simulink model "sensor_model"  (R2018a)
settings: Solver=VariableStepAuto  StartTime=0.0  StopTime=35  RelTol=1e-3
libraries: simulink x6
settings Model: Creator=cory0  LastModifiedBy=calvink

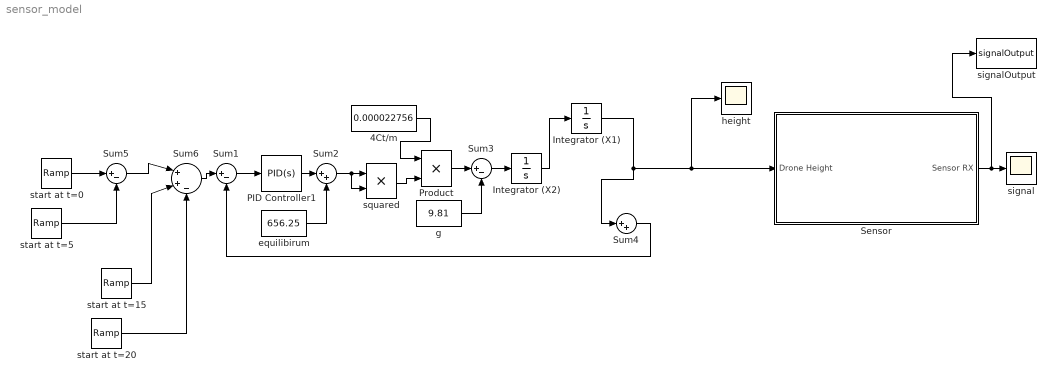
== system sensor_model ==
  4Ct/m : Constant  Value=0.000022756
  Integrator (X1) : Integrator
  Integrator (X2) : Integrator
  PID Controller1 : simulink/Continuous/PID Controller  Controller=PID  TimeDomain=Continuous-time  SampleTime=-1  IntegratorMethod=Forward Euler  FilterMethod=Forward Euler  Form=Parallel  UseFilter=on  ControllerParametersSource=internal  P=12.05  I=0  D=90  N=10  InitialConditionSource=internal  InitialConditionForIntegrator=0  InitialConditionForFilter=0  ExternalReset=none  LimitOutput=off  UpperSaturationLimit=inf  LowerSaturationLimit=-inf  LinearizeAsGain=on  AntiWindupMode=none  Kb=1  TrackingMode=off  Kt=1  PParamMin=[]  PParamMax=[]  IParamMin=[]  IParamMax=[]  DParamMin=[]  DParamMax=[]  NParamMin=[]  NParamMax=[]  KbParamMin=[]  KbParamMax=[]  KtParamMin=[]  KtParamMax=[]  POutMin=[]  POutMax=[]  IOutMin=[]  IOutMax=[]  DOutMin=[]  DOutMax=[]  NOutMin=[]  NOutMax=[]  KbOutMin=[]  KbOutMax=[]  KtOutMin=[]  KtOutMax=[]  IntegratorOutMin=[]  IntegratorOutMax=[]  FilterOutMin=[]  FilterOutMax=[]  SumOutMin=[]  SumOutMax=[]  SumI1OutMin=[]  SumI1OutMax=[]  SumI2OutMin=[]  SumI2OutMax=[]  SumI3OutMin=[]  SumI3OutMax=[]  SumDOutMin=[]  SumDOutMax=[]  SaturationOutMin=[]  SaturationOutMax=[]  IntegratorContinuousStateAttributes=''  IntegratorStateMustResolveToSignalObject=off  IntegratorRTWStateStorageClass=Auto  FilterContinuousStateAttributes=''  FilterStateMustResolveToSignalObject=off  FilterRTWStateStorageClass=Auto  DifferentiatorICPrevScaledInput=0  DifferentiatorOutMin=[]  DifferentiatorOutMax=[]  FilterDiffOutCoefMin=[]  FilterDiffOutCoefMax=[]  SumDenOutMin=[]  SumDenOutMax=[]  SumNumOutMin=[]  SumNumOutMax=[]  ReciprocalOutMin=[]  ReciprocalOutMax=[]  DivideOutMin=[]  DivideOutMax=[]  TunerSelectOption=Transfer Function Based (PID Tuner App)
  Product : Product
  Sensor : Subsystem
  Sum1 : Sum  Inputs=|+-
  Sum2 : Sum  Inputs=|++
  Sum3 : Sum  Inputs=|+-
  Sum4 : Sum  Inputs=|++
  Sum5 : Sum  Inputs=|+-
  Sum6 : Sum  Inputs=|++-
  equilibirum : Constant  Value=656.25
  g : Constant  Value=9.81
  height : Scope
  signal : Scope
  signalOutput : ToFile  Filename=signalOutput  MatrixName=raw
  squared : Product
  start at t=0 : simulink/Sources/Ramp  slope=1  start=0  InitialOutput=0
  start at t=15 : simulink/Sources/Ramp  slope=1  start=15  InitialOutput=0
  start at t=20 : simulink/Sources/Ramp  slope=1  start=20  InitialOutput=0
  start at t=5 : simulink/Sources/Ramp  slope=1  start=5  InitialOutput=0
  wires:
  Sensor/1(Sensor RX) -> signalOutput/1, signal/1
  Integrator (X2)/1 -> Integrator (X1)/1
  4Ct/m/1 -> Product/1
  Product/1 -> Sum3/1
  equilibirum/1 -> Sum2/2
  Sum3/1 -> Integrator (X2)/1
  Sum1/1 -> PID Controller1/1
  Sum2/1 -> squared/2, squared/1
  g/1 -> Sum3/2
  Integrator (X1)/1 -> height/1, Sensor/1(Drone Height), Sum4/1
  squared/1 -> Product/2
  Sum4/1 -> Sum1/2
  PID Controller1/1 -> Sum2/1
  start at t=0/1 -> Sum5/1
  start at t=5/1 -> Sum5/2
  start at t=20/1 -> Sum6/3
  start at t=15/1 -> Sum6/2
  Sum5/1 -> Sum6/1
  Sum6/1 -> Sum1/1

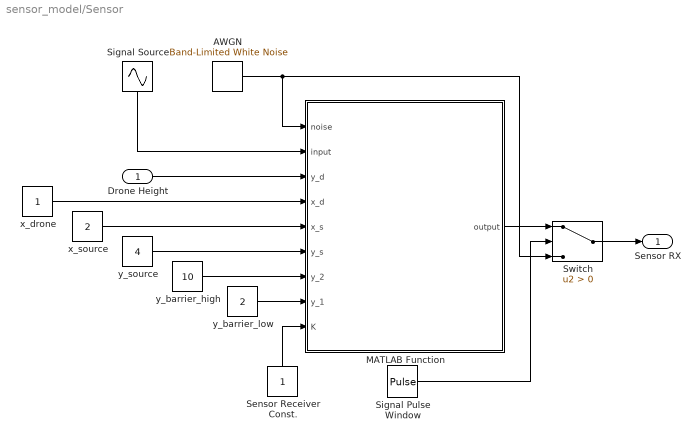
== system sensor_model/Sensor ==
  Drone Height : Inport
  AWGN : simulink/Sources/Band-Limited White Noise  Cov=[0.00001]  Ts=0.0005  seed=[23340]
  MATLAB Function : MATLAB Function  TreatAsAtomicUnit=on
  Sensor Receiver Const. : Constant
  Signal Source : Sin  Amplitude=10  Frequency=6.2831853  SampleTime=0
  Signal Pulse Window : DiscretePulseGenerator  PulseType=Time based  Period=20  PulseWidth=75
  Switch : Switch  Criteria=u2 > Threshold
  x_drone : Constant
  x_source : Constant  Value=2
  y_barrier_high : Constant  Value=10
  y_barrier_low : Constant  Value=2
  y_source : Constant  Value=4
  Sensor RX : Outport
  wires:
  Sensor Receiver Const./1 -> MATLAB Function/9(K)
  Signal Source/1 -> MATLAB Function/2(input)
  Signal Pulse Window/1 -> Switch/2
  y_source/1 -> MATLAB Function/6(y_s)
  y_barrier_low/1 -> MATLAB Function/8(y_1)
  x_drone/1 -> MATLAB Function/4(x_d)
  MATLAB Function/1(output) -> Switch/1
  AWGN/1 -> MATLAB Function/1(noise), Switch/3
  y_barrier_high/1 -> MATLAB Function/7(y_2)
  x_source/1 -> MATLAB Function/5(x_s)
  Drone Height/1 -> MATLAB Function/3(y_d)
  Switch/1 -> Sensor RX/1

== matlab function sensor_model/Sensor/MATLAB Function ==
  data: noise input; input input; y_d input; x_d input; output output; x_s input; y_s input; y_2 input; y_1 input; K input
function output = sensor_filter(noise,input,y_d,x_d,x_s,y_s,y_2,y_1,K)
    
    % Line of Sight Aperture
    c = y_d + (y_s-y_d)*x_d/(x_s+x_d);
    
    % Drone-Sensor Distance
    d = sqrt((x_d+x_s)^2 + (y_d-y_s)^2);
    
    % Sensor Reading
    if (c >= y_1) && (c <= y_2)
        output = sqrt(K)*input/d + noise;
    else
        output = noise;
    end

end
